simulink model "astron_hw_test_au50_64k"  (R2021a)
settings: Solver=VariableStepDiscrete  StartTime=0.0  StopTime=2048  RelTol=1e-3
undefined symbols (not defined in the file): d0, d1, d2, d3, FFT, sr, Wideband_FFT
libraries: xbsIndex_r4 x637, casper_library_misc x4, xps_library x1
(part 5 of 14)

== system astron_hw_test_au50_64k/bram_in3 ==
  addr : Inport
  data_in : Inport  Port=2
  we : Inport  Port=3
  Terminator : Terminator
  Terminator1 : Terminator
  Terminator2 : Terminator
  astron_hw_test_au50_64k_bram_in3_addr : xbsIndex_r4/Gateway Out  inherit_from_input=off  hdl_port=on  rows=1  columns=1  UseAsDAC=off  DACChannel='1'  interface=None  automatic_assignment=on  address_offset=hex2dec('00')  intf_name=''  intf_description=''  timing_constraint=None  locs_specified=off  LOCs={'A5','B9','A9','C1','A3','G6','E9','A6','A7','A8','B8','B1','B3','D9','B5','B4','B6','C2'}  io_standard={}  block_type=gatewayout
      settings: infoedit="Gateway out block.  Converts Xilinx fixed point inputs into ouputs of type Simulink integer, double, or fixed point.<P><P>Hardware notes:  In hardware these blocks become top level output ports or are discarded, depending on how they are configured."  sginterface={'Nallatech'=>{'xdspkit'=>{'non_memory_mapped_port'=>'uprev_Shared_BRAM_addr'}},'Xilinx'=>{'jtaghwcosim'=>{'non_memory_mapped_port'=>'uprev_Shared_BRAM_addr'},'xdspkit'=>{'non_memory_mapped_port'=>'uprev_Shared_BRAM_addr'}}}  xl_area=[0, 0, 0, 0, 0, 0, 0]
  astron_hw_test_au50_64k_bram_in3_data_in : xbsIndex_r4/Gateway Out  inherit_from_input=off  hdl_port=on  rows=1  columns=1  UseAsDAC=off  DACChannel='1'  interface=None  automatic_assignment=on  address_offset=hex2dec('00')  intf_name=''  intf_description=''  timing_constraint=None  locs_specified=off  LOCs={'B21','B22','A22','B23','B19','C19','A20','A21','A23','B24','A24','A25','E18','D18','C18','B18'}  io_standard={}  block_type=gatewayout
      settings: infoedit="Gateway out block.  Converts Xilinx fixed point inputs into ouputs of type Simulink integer, double, or fixed point.<P><P>Hardware notes:  In hardware these blocks become top level output ports or are discarded, depending on how they are configured."  sginterface={'Nallatech'=>{'xdspkit'=>{'non_memory_mapped_port'=>'uprev_Shared_BRAM_data_in'}},'Xilinx'=>{'jtaghwcosim'=>{'non_memory_mapped_port'=>'uprev_Shared_BRAM_data_in'},'xdspkit'=>{'non_memory_mapped_port'=>'uprev_Shared_BRAM_data_in'}}}  xl_area=[0, 0, 0, 0, 0, 0, 0]
  astron_hw_test_au50_64k_bram_in3_data_out : xbsIndex_r4/Gateway In  gui_display_data_type=Fixed-point  arith_type=Unsigned  n_bits=32  bin_pt=0  preci_type=Single  exp_width=8  frac_width=24  rows=1  columns=1  quantization=Truncate  overflow=Wrap  period=sample_rate  UseAsADC=off  ADCChannel='1'  interface=None  automatic_assignment=on  address_offset=hex2dec('00')  intf_name=''  intf_description=''  default_value=0  timing_constraint=None  locs_specified=off  LOCs={}  io_standard={}  inherit_from_input=off  hdl_port=on  dbl_ovrd=off  block_type=gatewayin
      settings: xl_area=[0, 0, 0, 0, 0, 0, 0]
  astron_hw_test_au50_64k_bram_in3_we : xbsIndex_r4/Gateway Out  inherit_from_input=off  hdl_port=on  rows=1  columns=1  UseAsDAC=off  DACChannel='1'  interface=None  automatic_assignment=on  address_offset=hex2dec('00')  intf_name=''  intf_description=''  timing_constraint=None  locs_specified=off  LOCs={'A14'}  io_standard={}  block_type=gatewayout
      settings: infoedit="Gateway out block.  Converts Xilinx fixed point inputs into ouputs of type Simulink integer, double, or fixed point.<P><P>Hardware notes:  In hardware these blocks become top level output ports or are discarded, depending on how they are configured."  xl_area=[0, 0, 0, 0, 0, 0, 0]
  calc_add : Subsystem  mask{data_width=32, addr_width=14, sample_rate=sample_rate}
      mask prompts: data_width "data width"; addr_width "address width"; sample_rate "sample rate"
  convert_addr : xbsIndex_r4/Convert  gui_display_data_type=Fixed-point  arith_type=Unsigned  n_bits=addr_width  bin_pt=0  float_type=Single  exp_bits=8  fraction_bits=24  quantization=Truncate  overflow=Wrap  en=off  latency=0  pipeline=off  dbl_ovrd=off  block_type=convert
      settings: xl_area=[0, 0, 0, 0, 0, 0, 0]
  convert_din1 : xbsIndex_r4/Convert  gui_display_data_type=Fixed-point  arith_type=Unsigned  n_bits=32  bin_pt=0  float_type=Single  exp_bits=8  fraction_bits=24  quantization=Truncate  overflow=Wrap  en=off  latency=0  pipeline=off  dbl_ovrd=off  block_type=convert
      settings: xl_area=[0, 0, 0, 0, 0, 0, 0]
  convert_we : xbsIndex_r4/Convert  gui_display_data_type=Fixed-point  arith_type=Unsigned  n_bits=1  bin_pt=0  float_type=Single  exp_bits=8  fraction_bits=24  quantization=Truncate  overflow=Wrap  en=off  latency=0  pipeline=off  dbl_ovrd=off  block_type=convert
      settings: xl_area=[0, 0, 0, 0, 0, 0, 0]
  munge_in : Subsystem  AncestorBlock=casper_library_flow_control/munge  mask(munge){divisions=1, div_size=32, order=[0], arith_type_out=Unsigned, bin_pt_out=0}
      mask prompts: divisions "Number of divisions"; div_size "Division size (bits)"; order "Division packing order"; arith_type_out "Output arithmetic type"; bin_pt_out "Output binary point"
      mask help: Splits an input bus into the specified number of divisions and then recombines them in the order specified (most significant division = 0,least = number divisions-1)
      mask init:
      | munge_init(gcb, ...
      |     'divisions', divisions, ...
      |     'div_size', div_size, ...
      |     'order', order, ...
      |     'arith_type_out', arith_type_out, ...
      |     'bin_pt_out', bin_pt_out);
      settings: AttributesFormatString=|
      | split:32
      | join:0
      | Unsigned [32,0]
      mask TypeOptions arith_type_out: Unsigned | Signed  (2's comp) | Floating-point
  munge_out : Subsystem  AncestorBlock=casper_library_flow_control/munge  mask(munge){divisions=1, div_size=32, order=[0], arith_type_out=Signed  (2's comp), bin_pt_out=0}
      mask prompts: divisions "Number of divisions"; div_size "Division size (bits)"; order "Division packing order"; arith_type_out "Output arithmetic type"; bin_pt_out "Output binary point"
      mask help: Splits an input bus into the specified number of divisions and then recombines them in the order specified (most significant division = 0,least = number divisions-1)
      mask init:
      | munge_init(gcb, ...
      |     'divisions', divisions, ...
      |     'div_size', div_size, ...
      |     'order', order, ...
      |     'arith_type_out', arith_type_out, ...
      |     'bin_pt_out', bin_pt_out);
      settings: AttributesFormatString=|
      | split:32
      | join:0
      | Signed  (2's comp) [32,0]
      mask TypeOptions arith_type_out: Unsigned | Signed  (2's comp) | Floating-point
  sim_mem : Subsystem  mask{arith_type=Signed  (2's comp), addr_width=14, data_width=32, data_bin_pt=0, init_vals=[9831  -2421  -6047   4171   1111   2206  -1845  -4827    944   1367    479   2297  -1311  -2137  -4696   2927  10466  -2954   2542  -7174   1296    905  -5528   1997   5032  -3841   9085  -3265  -9007   3587   3196  -7786   1045    232  -2612   1247   4431    556   2747  -3806    701  10149  -2394   4852   4649   2955   7953   -476   7611   5662  -2438    -21    653  -5045  -7011   4604   6485    771  -8623     40   2524    322  -5311  -2100   5832   -352   3592  -4387   -951  -1228  -3611  -1220   -666    863  -3316    198    239  -4951  -2256   1237  -3089   5232   3750   7107  -4638  -2435   2874   -952   3427  -3669  -1997   2995   9115   9164   1935  -1716   4089  -3093 -10713  -2793   4822    175   2154  -1206    279   4245   5735   1723   6850   5882   -832  -2450   -441   -902  -4702   3664  -6341  -2977    514   2690   3095  -2819   -604   1084   4622   9628    495   3322   7543   1572  -1649    497   5852   6250  -3513    -11  -1426   4728   5023   1431   3080   1744   5056  -1482  12109  -5280   2829  -1218    -89  -2719  -1958   3030  -1635   5098   -882   3625   8086   6964   4095   4210   5011  -8258  -5808   2237    892  -5280  -5959   4665   3390   2337   3640  -2781   4469  -2357   5622   8850    600   5417  -6979    774   -735   3776  -1172   -351   3021   3787  -2489   1513    -10   -536 -10282  -8660  -7018   5393 -14437  -1050   3342   -131    918  -4114   4893   1534  -8173  -3585   4321   4401   8999  -8078   1488  -4574  -7407   4966   5292  -2716  -5466   5971   8451   4520   -385   4484   1054  -3634   1231  -2774   9655  -9313  -6940    421  -2235   -264  -3834  -8002   2601   -734  -2170    217   5686    753  -1603  -4642   5214   -837   3496  -4884   2809  -2411   3538   4936     95   2883  -3789   -633   1812    376   -759   1631   6389   3980   5558   1443   3719  -2891  -1679   -601  -3442   4323   3537   -501   1698   -384  -5286    634    545  -2606    375  -1099   2542   4105  -2227   4054   3925    497   2425   4352   1058  -3139   5149   5384   5431    558   -340  -4447    165   1983  -8569   4400   3002   2297  -7189   1473   2921   5227   7702  -2987  10866  -1617   1098  -6489   2719   7481  -6821  -4489   5714  -2959   2275   1459  -2093   1429  -2390   1146   3583   4891   1045  -4476   3029   -690  -5013    380   2806   5316   4201  -4774   -826   2156   4473  -4181   1926   1674   3197   2879   2662   3569  -5326  -6544   -132  -3503  -7657   3030   6141   1867  -3966   7463   1085  -4343   4296  -1524   2972    664     60  -6092   2145   3939   3502    499    -45  -1874   -413   1848   -959   1391  -8354   2708   5105   4712  -1323  -1891 -10075  -5460  -3461    847   4303   3888  -2691  -7305   2921   4445   2691   -407   2602    315  -4447   5599   2141   -317   8240  -2487   2358  -3737  -1447  -2070   4984   3040  -4375   3305   7550   3862  -4944   4744  -4384   4160  -9436  -4826   2974  -2059  -2464  -1430   4849  -2439  -3601  -9037    -81   2945  -2469  -9267  11803   3373   3804  -3081    -66   -500  -9192  -8934   8238  -2864  -2284   1172   6592   2001  -4265  10914   3099   6501  -6350  -3752   3474  -4081  -1622   1572  -2254   2453  -3545    467  -4155   5924  -5390   1283   4483  -1342   1566   -686  -1045   1909  -8853   -259   -741   7246  -3638  -6871   4152  -1593   9605   -750    557   3795  -9120    911   -787    720  -1927  -5429    850   6027  -1036    813  10537  -4523  -4090   2963   3719   4193  -3434  -6675  12818    530  -2443   -837   4345   -531  -2115  -7538  -2682   5450   1417   -667   2999  -2980   -762  -1589  -3818     79   8830    944   5004  -1188    283   2023   4847  -2111    593  -1129   7089   3923   5204   5749  -3732    479  -9948   2568   7734  -2288  -8598   1855  -1826   1832  -6373   1361   2929   5173  -6636  -8558   8898  -2237  -6733  -5095   2805    718   -596   1020  -5987  -1028  -4944  -6752   7847  10132    510  -1457   1205   5056   3500   5474    382   1127   -598  -6182    -97   2599  -4652  -4276   1154  -3994   -953 ...(+110690 chars)], sample_rate=1, csp_latency=1}
      mask prompts: arith_type "Output Data Type"; addr_width "Address width"; data_width "Data width"; data_bin_pt "Data Binary Point"; init_vals "Initial values"; sample_rate "Sample rate"; csp_latency "Latency"
      mask init:
      | % set_param([gcb, '/data_to_xilinx'], 'arith_type', arith_type)
      | % set_param([gcb, '/data_to_xilinx'], 'n_bits', get_param(gcb, 'data_width'))
      mask TypeOptions arith_type: Unsigned | Signed  (2's comp)
      mask TypeOptions data_width: 8 | 16 | 32 | 64 | 128
  data_out : Outport  VectorParamsAs1DForOutWhenUnconnected=off
  wires:
  munge_out/1(dout) -> data_out/1
  sim_mem/1(data_out) -> astron_hw_test_au50_64k_bram_in3_data_out/1
  astron_hw_test_au50_64k_bram_in3_data_out/1 -> munge_out/1(din)
  convert_addr/1 -> astron_hw_test_au50_64k_bram_in3_addr/1
  convert_din1/1 -> astron_hw_test_au50_64k_bram_in3_data_in/1
  data_in/1 -> munge_in/1(din)
  calc_add/1(out) -> convert_addr/1
  astron_hw_test_au50_64k_bram_in3_we/1 -> Terminator2/1
  astron_hw_test_au50_64k_bram_in3_data_in/1 -> Terminator1/1
  astron_hw_test_au50_64k_bram_in3_addr/1 -> Terminator/1
  convert_we/1 -> astron_hw_test_au50_64k_bram_in3_we/1
  addr/1 -> sim_mem/1(addr), calc_add/1(in)
  we/1 -> sim_mem/3(we), convert_we/1
  munge_in/1(dout) -> sim_mem/2(data), convert_din1/1
